simulink model "Simulation"  (R2020a)
settings: Solver=VariableStepAuto  StartTime=0.0  StopTime=15  RelTol=1e-3
values from neighbouring files (symbols this model uses):
  AirDensity = 1.225    [ThrustData.m]
  Area = pi*(0.02)^2    (= 0.00125663706144)    [ThrustData.m]
  DragCoef = 0.75    [ThrustData.m]
  EngineMass = 0.0258    [ThrustData.m]
  EngineThrust = data(:,2)    [ThrustData.m]
  PropMass = 0.0108    [ThrustData.m]
  RocketMass = 0.1    [ThrustData.m]
  ThrustTime = data(:,1)    [ThrustData.m]
  TotalImpulse = 8.817    [ThrustData.m]
settings Model: Creator=user  LastModifiedBy=user

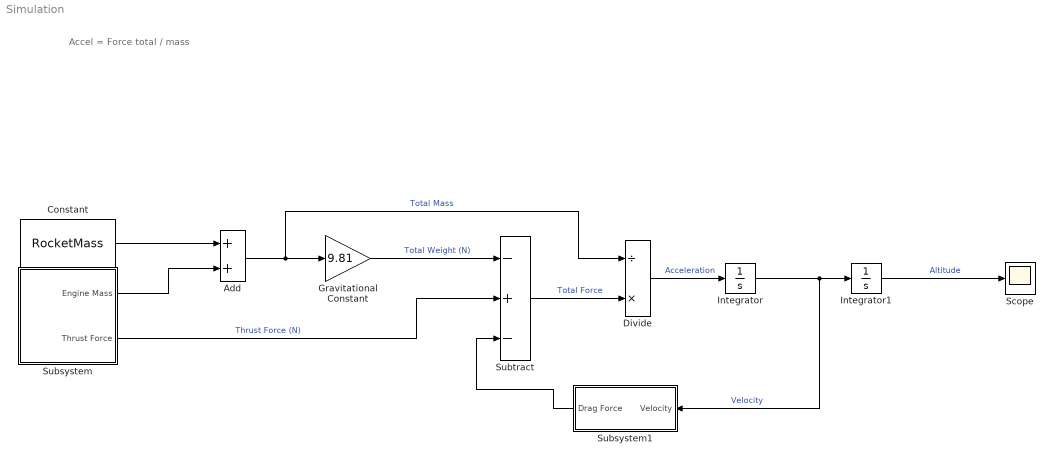
== system Simulation ==
  note: Accel = Force total / mass
  Add : Sum
  Constant : Constant  Value=RocketMass
  Divide : Product  Inputs=/*
  Gravitational Constant : Gain  Gain=9.81
  Integrator : Integrator  LimitOutput=on
  Integrator1 : Integrator  LimitOutput=on  LowerSaturationLimit=0
  Scope : Scope
  Subsystem : Subsystem
  Subsystem1 : Subsystem
  Subtract : Sum  Inputs=-+-
  wires:
  Constant/1 -> Add/1
  Add/1 -> Divide/1, Gravitational Constant/1  "Total Mass"
  Gravitational Constant/1 -> Subtract/1  "Total Weight (N)"
  Subsystem/1(Engine Mass) -> Add/2
  Subsystem/2(Thrust Force) -> Subtract/2  "Thrust Force (N)"
  Subtract/1 -> Divide/2  "Total Force"
  Divide/1 -> Integrator/1  "Acceleration"
  Integrator/1 -> Subsystem1/1(Velocity), Integrator1/1  "Velocity"
  Subsystem1/1(Drag Force) -> Subtract/3
  Integrator1/1 -> Scope/1  "Altitude"

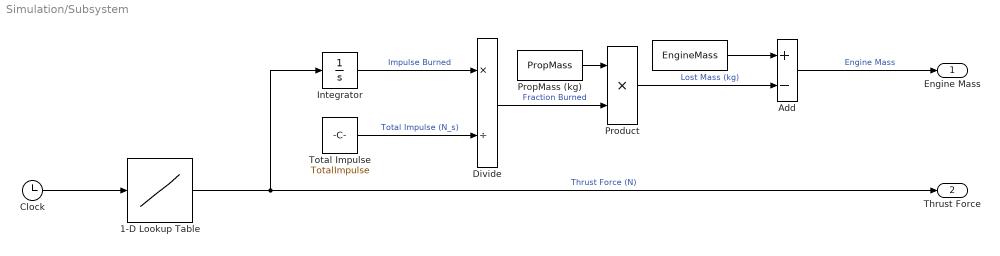
== system Simulation/Subsystem ==
  " " : Constant  Value=EngineMass
  1-D Lookup Table : Lookup_n-D  NumberOfTableDimensions=1  BreakpointsForDimension1=ThrustTime  Table=EngineThrust  InternalRulePriority=Speed  RndMeth=Simplest  InputSameDT=on
  Add : Sum  Inputs=+-
  Clock : Clock
      settings: Decimation=15
  Divide : Product  Inputs=*/
  Integrator : Integrator
  Product : Product
  PropMass (kg) : Constant  Value=PropMass
  Total Impulse : Constant  Value=TotalImpulse
  Engine Mass : Outport
  Thrust Force : Outport  Port=2
  wires:
  Add/1 -> Engine Mass/1  "Engine Mass"
  Total Impulse/1 -> Divide/2  "Total Impulse (N_s)"
  Integrator/1 -> Divide/1  "Impulse Burned"
  Clock/1 -> 1-D Lookup Table/1
  PropMass (kg)/1 -> Product/1
  1-D Lookup Table/1 -> Thrust Force/1, Integrator/1  "Thrust Force (N)"
  " "/1 -> Add/1
  Product/1 -> Add/2  "Lost Mass (kg)"
  Divide/1 -> Product/2  "Fraction Burned"

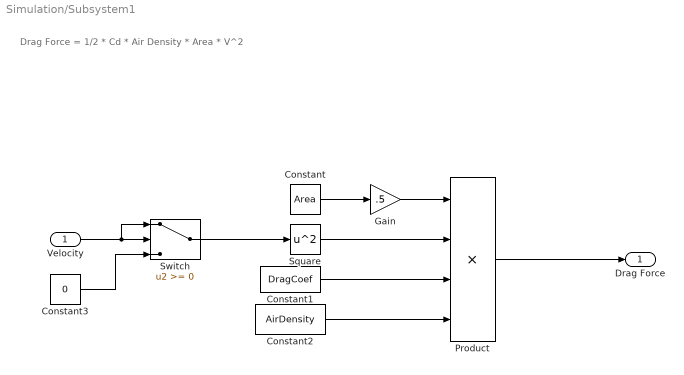
== system Simulation/Subsystem1 ==
  note: Drag Force = 1/2 * Cd * Air Density * Area * V^2
  Velocity : Inport
  Constant : Constant  Value=Area
  Constant1 : Constant  Value=DragCoef
  Constant2 : Constant  Value=AirDensity
  Constant3 : Constant  Value=0
  Gain : Gain  Gain=.5
  Product : Product  Inputs=4
  Square : Math  Operator=square  SaturateOnIntegerOverflow=on
  Switch : Switch
  Drag Force : Outport
  wires:
  Velocity/1 -> Switch/1, Switch/2
  Constant/1 -> Gain/1
  Square/1 -> Product/2
  Gain/1 -> Product/1
  Constant1/1 -> Product/3
  Constant2/1 -> Product/4
  Product/1 -> Drag Force/1
  Switch/1 -> Square/1
  Constant3/1 -> Switch/3
